simulink model "Load_Rate_Actuator"  (R2012b)
settings: Solver=ode4  StartTime=0.0  StopTime=2.999  FixedStep=1e-5  MaxStep=1e-3  MinStep=1e-4
undefined symbols (not defined in the file or in its folder): Acv, Aleak1, Aleak2, Aleak3, Aleak4, Aleak5, Aleakext, Aleakint, Ap, Ap_seal, Ar_seal, As_ehsv, Bkp_seal, Bp1, C, Cd, DeltaQ_ehsv, EHSV, EHSV_step, EHSVFreqTest, EHSVTest, ent_air, frictionstribeck_velocity, i_ehsv, K2_ehsv, K3_ehsv, K_Supply1, Ka1, Ki_ehsv, Kr_ehsv, ksi_ehsv, Kst, Kst_Enable, Kw_ehsv, L0, load_cmd, Lp_seal, Lr_seal, Mp1, P10, Pcvac, Pcvi, Pcvr, Ps0, Pt0, Ql_ehsv, R, rate_high, rate_low, Return_Pressure, Rho, seal_compression, seal_hardness, SealConstValue, SealType, Supply_Pressure, Temp, Theta0, V011, V021 ... (+10)
undefined symbols (not defined in the file): dpLVDT, ramLVDT, xvLVDT
libraries: simulink x2
(part 1 of 2)
settings Model: SimulationMode=accelerator  Creator=Charles  LastModifiedBy=hballest
settings SolverCC: InitialStep=1e-4
settings DataIOCC: LimitDataPoints=off  SaveFormat=StructureWithTime  DSMLogging=off  SaveTime=off
settings OptimizationCC: InitFltsAndDblsToZero=on
settings DebuggingCC: SaveWithParameterizedLinksMsg=none  InheritedTsInSrcMsg=none  FcnCallInpInsideContextMsg=UseLocalSettings  LoggingUnavailableSignals=none
settings ModelReferenceCC: UpdateModelReferenceTargets=IfOutOfDate
settings GRTTargetCC: TargetFcnLib=ansi_tfl_tmw.mat  CombineOutputUpdateFcns=off  GRTInterface=on

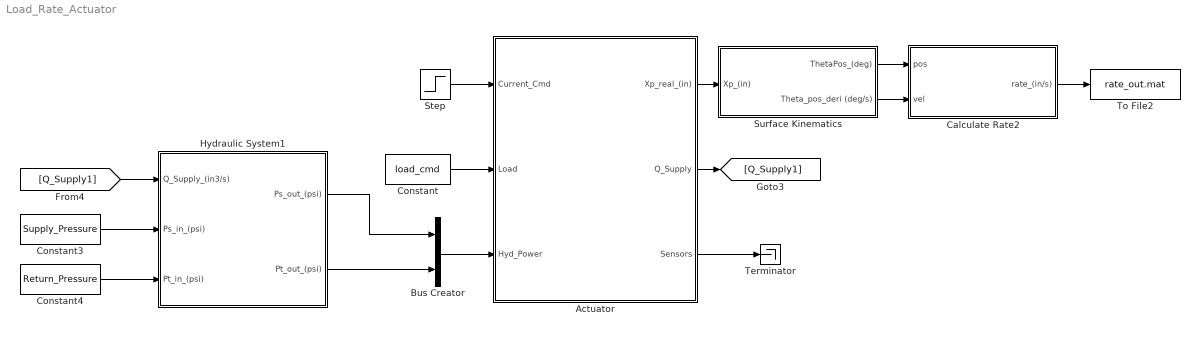
== system Load_Rate_Actuator ==
  Actuator : Subsystem
  Bus Creator : BusCreator  Inputs=2
  Calculate Rate2 : Subsystem
  Constant : Constant  Value=load_cmd
  Constant3 : Constant  Value=Supply_Pressure
  Constant4 : Constant  Value=Return_Pressure
  Hydraulic System1 : Subsystem
  Step : Step  Time=.5  After=EHSV_step.final  SampleTime=0
  Surface Kinematics : Subsystem
  Terminator : Terminator
  To File2 : ToFile  Filename=rate_out.mat  MatrixName=rate_out
  wires:
  Actuator/1(Xp_real_(in)) -> Surface Kinematics/1(Xp_(in))
  Constant3/1 -> Hydraulic System1/2(Ps_in_(psi))
  Constant4/1 -> Hydraulic System1/3(Pt_in_(psi))
  Hydraulic System1/1(Ps_out_(psi)) -> Bus Creator/1
  Hydraulic System1/2(Pt_out_(psi)) -> Bus Creator/2
  [Q_Supply1] -> Hydraulic System1/1(Q_Supply_(in3/s))
  Bus Creator/1 -> Actuator/3(Hyd_Power)
  Actuator/2(Q_Supply) -> [Q_Supply1]
  Actuator/3(Sensors) -> Terminator/1
  Constant/1 -> Actuator/2(Load)
  Step/1 -> Actuator/1(Current_Cmd)
  Surface Kinematics/1(ThetaPos_(deg)) -> Calculate Rate2/1(pos)
  Surface Kinematics/2(Theta_pos_deri (deg/s)) -> Calculate Rate2/2(vel)
  Calculate Rate2/1(rate_(in/s)) -> To File2/1

== system Load_Rate_Actuator/Actuator ==
  Current_Cmd : Inport
  Load : Inport  Port=2
  Hyd_Power : Inport  Port=3
  Cylinder Dynamics : Subsystem
  Sensors Dynamics : Subsystem
  Valves Dynamics : Subsystem
  Xp_real_(in) : Outport
  Q_Supply : Outport  Port=2
  Sensors : Outport  Port=3
  wires:
  Cylinder Dynamics/2(Xp) -> [Xp], Xp_real_(in)/1
  Load/1 -> Cylinder Dynamics/2(Load)
  Valves Dynamics/2(Q_Supply) -> Q_Supply/1
  Valves Dynamics/1(Q_Act) -> Cylinder Dynamics/1(Q_Act)
  Current_Cmd/1 -> Valves Dynamics/2(Currrent)
  Hyd_Power/1 -> Valves Dynamics/3(Hyd_Pwr)
  Cylinder Dynamics/1(P_Act) -> Valves Dynamics/1(P_Act)
  Cylinder Dynamics/3(Qacv) -> Valves Dynamics/4(Qacv)
  Valves Dynamics/3(Pt) -> Cylinder Dynamics/3(Pt)
  Valves Dynamics/4(Xv_(in)) -> [Xv]
  Cylinder Dynamics/4(dP) -> [dP]
  [Xp] -> Sensors Dynamics/1(Xp)
  [dP] -> Sensors Dynamics/2(dP)
  [Xv] -> Sensors Dynamics/3(Xv)
  Sensors Dynamics/1(Sensors) -> Sensors/1

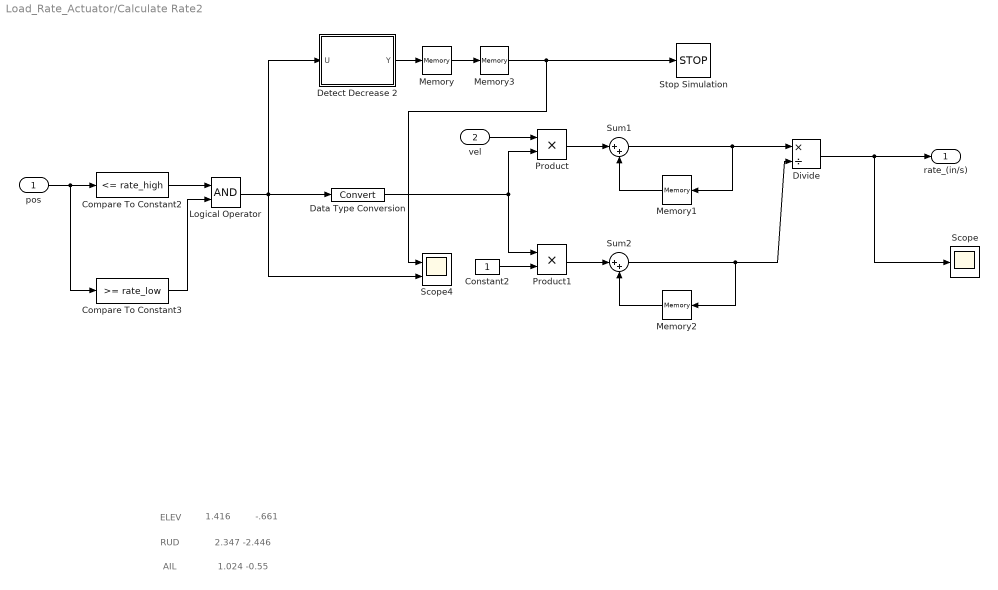
== system Load_Rate_Actuator/Calculate Rate2 ==
  note: 2.347 -2.446
  note: RUD
  note: ELEV
  note: -.661
  note: 1.416
  note: 1.024 -0.55
  note: AIL
  pos : Inport
  vel : Inport  Port=2
  Compare To Constant2 : simulink/Logic and Bit Operations/Compare To Constant  relop=<=  const=rate_high  OutDataTypeStr=boolean
  Compare To Constant3 : simulink/Logic and Bit Operations/Compare To Constant  relop=>=  const=rate_low  OutDataTypeStr=boolean
  Constant2 : Constant
  Data Type Conversion : DataTypeConversion
  Detect Decrease 2 : Subsystem
  Divide : Product  Inputs=*/
  Logical Operator : Logic  AllPortsSameDT=off  OutDataTypeStr=boolean
  Memory : Memory  X0=0.0
  Memory1 : Memory
  Memory2 : Memory  X0=0.0001
  Memory3 : Memory  X0=0.0
  Product : Product  RndMeth=Zero
  Product1 : Product  RndMeth=Zero
  Scope : Scope
      settings: SaveName=ScopeData5
  Scope4 : Scope  NumInputPorts=2
      settings: YMin=-5~-5  YMax=5~5  SaveName=ScopeData13
  Stop Simulation : Stop
  Sum1 : Sum  Inputs=|++
  Sum2 : Sum  Inputs=|++
  rate_(in/s) : Outport
  wires:
  pos/1 -> Compare To Constant2/1, Compare To Constant3/1
  Detect Decrease 2/1(Y) -> Memory/1
  Constant2/1 -> Product1/2
  Product1/1 -> Sum2/1
  Sum2/1 -> Memory2/1, Divide/2
  Memory2/1 -> Sum2/2
  Data Type Conversion/1 -> Product/2, Product1/1
  Compare To Constant3/1 -> Logical Operator/2
  Compare To Constant2/1 -> Logical Operator/1
  Sum1/1 -> Divide/1, Memory1/1
  Product/1 -> Sum1/1
  Memory1/1 -> Sum1/2
  vel/1 -> Product/1
  Logical Operator/1 -> Detect Decrease 2/1(U), Scope4/2, Data Type Conversion/1
  Memory/1 -> Memory3/1
  Memory3/1 -> Stop Simulation/1, Scope4/1
  Divide/1 -> Scope/1, rate_(in/s)/1

== system Load_Rate_Actuator/Hydraulic System1 ==
  Q_Supply_(in3/s) : Inport
  Ps_in_(psi) : Inport  Port=2
  Pt_in_(psi) : Inport  Port=3
  Aircraft Hydraulic Losses : Gain  Gain=K_Supply1
  Bus Selector : BusSelector  OutputSignals=Qs
  Fluid Inertia : TransferFcn  Denominator=[0.01 1]
  Sum1 : Sum  Inputs=|+-
  cis to gpm : Gain  Gain=0.25974
  Ps_out_(psi) : Outport
  Pt_out_(psi) : Outport  Port=2
  wires:
  Sum1/1 -> Ps_out_(psi)/1  "Ps"
  Aircraft Hydraulic Losses/1 -> Fluid Inertia/1
  Fluid Inertia/1 -> Sum1/2
  Pt_in_(psi)/1 -> Pt_out_(psi)/1  "Pt"
  Ps_in_(psi)/1 -> Sum1/1  "Ps"
  Q_Supply_(in3/s)/1 -> Bus Selector/1
  cis to gpm/1 -> Aircraft Hydraulic Losses/1
  Bus Selector/1 -> cis to gpm/1  "<Qs>"

== system Load_Rate_Actuator/Surface Kinematics ==
  Xp_(in) : Inport
  Derivative : Derivative
  Rad2Deg : Gain  Gain=180/pi  SaturateOnIntegerOverflow=on  OutDataTypeStr=Inherit: Same as input  ParamDataTypeStr=Inherit: Same as input
  Real Kinematics : Subsystem
  Terminator : Terminator
  ThetaPos_(deg) : Outport
  Theta_pos_deri (deg/s) : Outport  Port=2
  wires:
  Xp_(in)/1 -> Real Kinematics/1(Xp)
  Real Kinematics/1(Theta) -> Rad2Deg/1
  Rad2Deg/1 -> Derivative/1, ThetaPos_(deg)/1
  Real Kinematics/2(Reff) -> Terminator/1
  Derivative/1 -> Theta_pos_deri (deg/s)/1

== system Load_Rate_Actuator/Actuator/Cylinder Dynamics ==
  Q_Act : Inport
  Load : Inport  Port=2
  Pt : Inport  Port=3
  Bus Creator1 : BusCreator  Inputs=2
  Bus Creator3 : BusCreator  Inputs=2
  Bus Selector : BusSelector  OutputSignals=Q1,Q2
  Fluid Dynamics : Subsystem
  Piston Dynamics : Subsystem
  P_Act : Outport
  Xp : Outport  Port=2
  Qacv : Outport  Port=3
  dP : Outport  Port=4
  wires:
  Bus Creator3/1 -> P_Act/1
  Q_Act/1 -> Bus Selector/1
  Bus Selector/2 -> Fluid Dynamics/4(Q2)  "<Q2>"
  Piston Dynamics/1(Xp) -> [Xp], Xp/1
  Piston Dynamics/2(Xpdot) -> [Xpdot]  "Xpdot"
  [Xp] -> Fluid Dynamics/1(xp)
  [Xpdot] -> Fluid Dynamics/2(xpdot)
  Load/1 -> Piston Dynamics/3(FL)
  Bus Selector/1 -> Fluid Dynamics/3(Q1)  "<Q1>"
  Fluid Dynamics/2(P2) -> Piston Dynamics/2(Pr), Bus Creator3/2  "P2"
  Fluid Dynamics/1(P1) -> Piston Dynamics/1(Pe), Bus Creator3/1  "P1"
  Pt/1 -> Fluid Dynamics/5(Pt)
  Fluid Dynamics/3(Qacv1) -> Bus Creator1/1  "Qacv1"
  Fluid Dynamics/4(Qacv2) -> Bus Creator1/2  "Qacv2"
  Bus Creator1/1 -> Qacv/1
  Fluid Dynamics/5(dP) -> dP/1

== system Load_Rate_Actuator/Actuator/Sensors Dynamics ==
  Xp : Inport
  dP : Inport  Port=2
  Xv : Inport  Port=3
  Bus Creator : BusCreator  Inputs=3
  "Xp LVDT " : Subsystem
  "Xv LVDT " : Subsystem
  "dP LVDT " : Subsystem
  Sensors : Outport
  wires:
  dP/1 -> "dP LVDT "/1(dP_real)
  Xp/1 -> "Xp LVDT "/1(Xp_real)
  Xv/1 -> "Xv LVDT "/1(Xv_real)
  "Xv LVDT "/1(Xv_LVDT) -> Bus Creator/3  "Xv_mesured_(in)"
  "dP LVDT "/1(dP_LVDT) -> Bus Creator/2  "dP_mesured_(psi)"
  "Xp LVDT "/1(Xp_LVDT) -> Bus Creator/1  "Xp_mesured_(in)"
  Bus Creator/1 -> Sensors/1

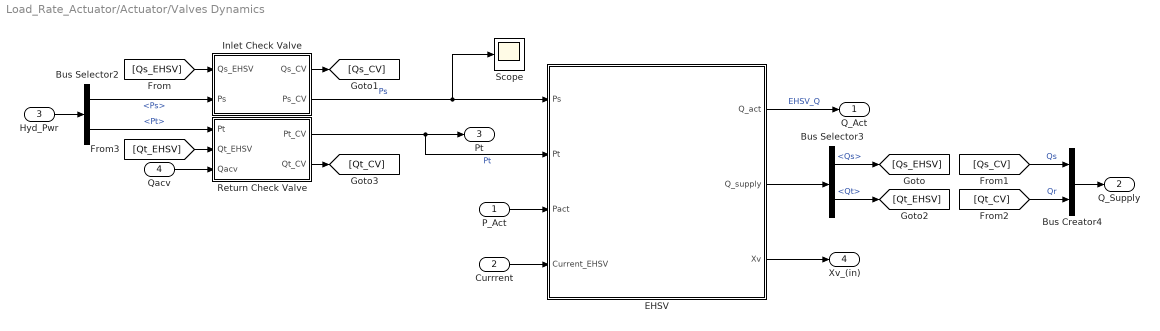
== system Load_Rate_Actuator/Actuator/Valves Dynamics ==
  P_Act : Inport
  Currrent : Inport  Port=2
  Hyd_Pwr : Inport  Port=3
  Qacv : Inport  Port=4
  Bus Creator4 : BusCreator  Inputs=2
  Bus Selector2 : BusSelector  OutputSignals=Ps,Pt
  Bus Selector3 : BusSelector  OutputSignals=Qs,Qt
  EHSV : Subsystem
  Inlet Check Valve : Subsystem
  Return Check Valve : Subsystem
  Scope : Scope
      settings: SaveName=ScopeData5
  Q_Act : Outport
  Q_Supply : Outport  Port=2
  Pt : Outport  Port=3
  Xv_(in) : Outport  Port=4
  wires:
  Hyd_Pwr/1 -> Bus Selector2/1
  EHSV/1(Q_act) -> Q_Act/1  "EHSV_Q"
  Bus Selector2/1 -> Inlet Check Valve/2(Ps)  "<Ps>"
  Bus Selector3/1 -> [Qs_EHSV]  "<Qs>"
  [Qs_EHSV] -> Inlet Check Valve/1(Qs_EHSV)
  Inlet Check Valve/1(Qs_CV) -> [Qs_CV]
  [Qs_CV] -> Bus Creator4/1  "Qs"
  Bus Creator4/1 -> Q_Supply/1
  Bus Selector2/2 -> Return Check Valve/1(Pt)  "<Pt>"
  Bus Selector3/2 -> [Qt_EHSV]  "<Qt>"
  [Qt_CV] -> Bus Creator4/2  "Qr"
  [Qt_EHSV] -> Return Check Valve/2(Qt_EHSV)
  Return Check Valve/2(Qt_CV) -> [Qt_CV]
  Qacv/1 -> Return Check Valve/3(Qacv)
  Currrent/1 -> EHSV/4(Current_EHSV)
  P_Act/1 -> EHSV/3(Pact)
  Inlet Check Valve/2(Ps_CV) -> Scope/1, EHSV/1(Ps)  "Ps"
  Return Check Valve/1(Pt_CV) -> EHSV/2(Pt), Pt/1  "Pt"
  EHSV/2(Q_supply) -> Bus Selector3/1
  EHSV/3(Xv) -> Xv_(in)/1

== system Load_Rate_Actuator/Calculate Rate2/Detect Decrease 2 ==
  note: Edge
  note: U(k)
  U : Inport
  FixPt Relational Operator : RelationalOperator  Operator=<  OutDataTypeStr=boolean  ZeroCross=off
  Memory : Memory  X0=0.0
  Y : Outport  InitialOutput=0
  wires:
  U/1 -> Memory/1, FixPt Relational Operator/1
  FixPt Relational Operator/1 -> Y/1
  Memory/1 -> FixPt Relational Operator/2  "U(k-1)"

== system Load_Rate_Actuator/Surface Kinematics/Real Kinematics ==
  Xp : Inport
  Bus Creator : BusCreator
  Bus Selector2 : BusSelector  OutputSignals=C,R,L
  Bus Selector3 : BusSelector  OutputSignals=L,C,R
  Bus Selector4 : BusSelector  OutputSignals=Theta0
  Bus Selector5 : BusSelector  OutputSignals=C
  Constant : Constant  Value=L0
  Constant1 : Constant  Value=R
  Constant2 : Constant  Value=C
  Constant3 : Constant  Value=Theta0
  Law of cosines Get angle : Fcn  Expr=acos((u(1)^2+u(2)^2-u(3)^2)/(2*u(1)*u(2)))
  Law of cosines Get angle1 : Fcn  Expr=acos((u(1)^2+u(2)^2-u(3)^2)/(2*u(1)*u(2)))
  Mux1 : Mux  Inputs=3
  Mux2 : Mux  Inputs=3
  Product : Product  RndMeth=Zero
  Sum1 : Sum  Inputs=++|
  Sum4 : Sum  Inputs=|+-
  Trigonometric Function : Trigonometry
  Theta : Outport
  Reff : Outport  Port=2
  wires:
  Mux2/1 -> Law of cosines Get angle1/1
  Bus Selector2/1 -> Mux2/1  "<C>"
  Bus Selector2/2 -> Mux2/2  "<R>"
  Law of cosines Get angle1/1 -> Sum4/1  "theta"
  Bus Selector4/1 -> Sum4/2  "<Theta0>"
  Sum4/1 -> Theta/1
  Xp/1 -> Sum1/1  "Xp"
  Constant/1 -> Sum1/2  "L0"
  Sum1/1 -> Bus Creator/1  "L"
  Constant2/1 -> Bus Creator/2  "C"
  Constant1/1 -> Bus Creator/3  "R"
  Constant3/1 -> Bus Creator/4  "Theta0"
  Mux1/1 -> Law of cosines Get angle/1
  Law of cosines Get angle/1 -> Trigonometric Function/1  "alfa"
  Bus Selector3/1 -> Mux1/1  "<L>"
  Bus Selector3/2 -> Mux1/2  "<C>"
  Bus Selector3/3 -> Mux1/3  "<R>"
  Product/1 -> Reff/1  "Reff"
  Bus Selector5/1 -> Product/1  "<C>"
  Trigonometric Function/1 -> Product/2
  Bus Selector2/3 -> Mux2/3  "<L>"
  Bus Creator/1 -> Bus Selector3/1, Bus Selector5/1, Bus Selector2/1, Bus Selector4/1

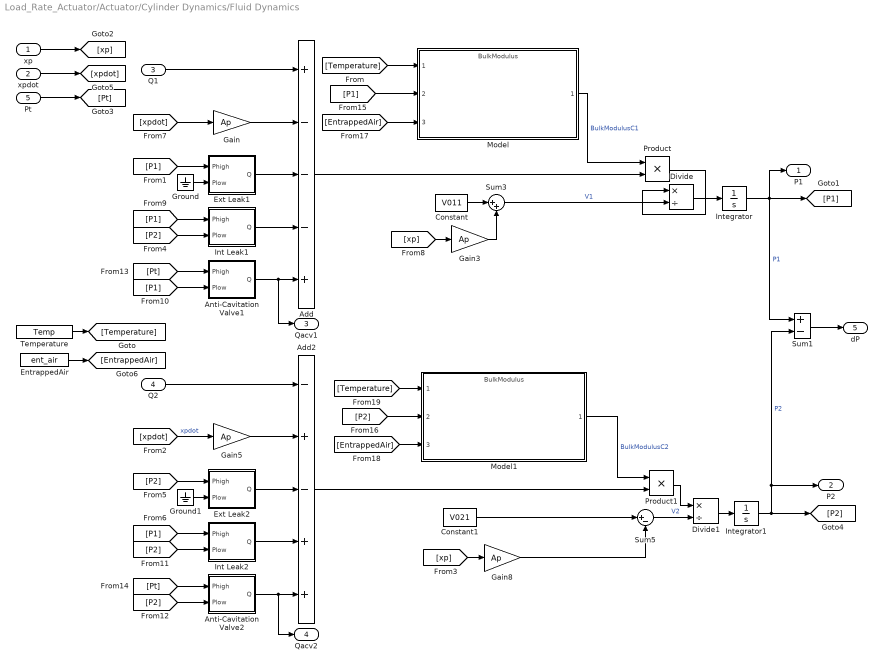
== system Load_Rate_Actuator/Actuator/Cylinder Dynamics/Fluid Dynamics ==
  xp : Inport
  xpdot : Inport  Port=2
  Q1 : Inport  Port=3
  Q2 : Inport  Port=4
  Pt : Inport  Port=5
  Add : Sum  Inputs=+---+
  Add2 : Sum  Inputs=-+-++
  Anti-Cavitation Valve1 : Subsystem
  Anti-Cavitation Valve2 : Subsystem
  Constant : Constant  Value=V011
  Constant1 : Constant  Value=V021
  Divide : Product  Inputs=*/
  Divide1 : Product  Inputs=*/
  EntrappedAir : Constant  Value=ent_air
  Ext Leak1 : Subsystem
  Ext Leak2 : Subsystem
  Gain{,3,5,8} (4 alike) : Gain  Gain=Ap
  Ground : Ground
  Ground1 : Ground
  Int Leak1 : Subsystem
  Int Leak2 : Subsystem
  Integrator : Integrator  InitialCondition=P10
  Integrator1 : Integrator  InitialCondition=P10
  Model : ModelReference  ModelNameDialog=BulkModulus  SimulationMode=Normal  ModelReferenceVersion=1.7  CopyOfModelName=BulkModulus  DefaultDataLogging=off
  Model1 : ModelReference  ModelNameDialog=BulkModulus  SimulationMode=Normal  ModelReferenceVersion=1.7  CopyOfModelName=BulkModulus  DefaultDataLogging=off
  Product : Product  RndMeth=Zero
  Product1 : Product  RndMeth=Zero
  Sum1 : Sum  Inputs=+-
  Sum3 : Sum  Inputs=|++
  Sum5 : Sum  Inputs=|+-
  Temperature : Constant  Value=Temp
  P1 : Outport
  P2 : Outport  Port=2
  Qacv1 : Outport  Port=3
  Qacv2 : Outport  Port=4
  dP : Outport  Port=5
  wires:
  Q1/1 -> Add/1
  Q2/1 -> Add2/1
  [xpdot] -> Gain5/1  "xpdot"
  [xp] -> Gain8/1
  Int Leak2/1(Q) -> Add2/4
  Divide1/1 -> Integrator1/1
  Sum5/1 -> Divide1/2  "V2"
  Gain8/1 -> Sum5/2
  Constant1/1 -> Sum5/1
  Integrator1/1 -> [P2], Sum1/2, P2/1  "P2"
  Ext Leak2/1(Q) -> Add2/3
  Gain5/1 -> Add2/2
  Int Leak1/1(Q) -> Add/4
  Divide/1 -> Integrator/1
  Sum3/1 -> Divide/2  "V1"
  Gain3/1 -> Sum3/2
  Constant/1 -> Sum3/1
  Integrator/1 -> Sum1/1, [P1], P1/1  "P1"
  Ext Leak1/1(Q) -> Add/3
  Add/1 -> Product/2
  Gain/1 -> Add/2
  [P1] -> Ext Leak1/1(Phigh)
  [P2] -> Ext Leak2/1(Phigh)
  xpdot/1 -> [xpdot]
  [xpdot] -> Gain/1
  xp/1 -> [xp]
  [xp] -> Gain3/1
  [P2] -> Int Leak1/2(Plow)
  Ground/1 -> Ext Leak1/2(Plow)
  Ground1/1 -> Ext Leak2/2(Plow)
  [P1] -> Int Leak2/1(Phigh)
  [Pt] -> Anti-Cavitation Valve1/1(Phigh)
  [P1] -> Anti-Cavitation Valve1/2(Plow)
  [P1] -> Int Leak1/1(Phigh)
  Anti-Cavitation Valve1/1(Q) -> Add/5, Qacv1/1
  [P2] -> Int Leak2/2(Plow)
  Anti-Cavitation Valve2/1(Q) -> Add2/5, Qacv2/1
  [Pt] -> Anti-Cavitation Valve2/1(Phigh)
  [P2] -> Anti-Cavitation Valve2/2(Plow)
  Pt/1 -> [Pt]
  Product/1 -> Divide/1
  [P1] -> Model/2
  Model/1 -> Product/1  "BulkModulusC1"
  Product1/1 -> Divide1/1
  Model1/1 -> Product1/1  "BulkModulusC2"
  Add2/1 -> Product1/2
  [P2] -> Model1/2
  Temperature/1 -> [Temperature]
  EntrappedAir/1 -> [EntrappedAir]
  [Temperature] -> Model/1
  [EntrappedAir] -> Model/3
  [EntrappedAir] -> Model1/3
  [Temperature] -> Model1/1
  Sum1/1 -> dP/1

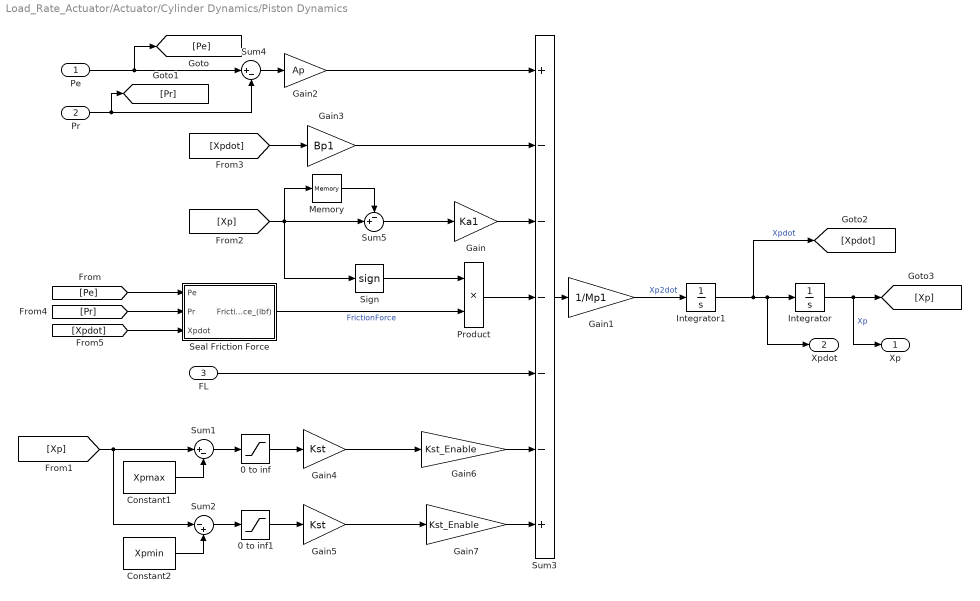
== system Load_Rate_Actuator/Actuator/Cylinder Dynamics/Piston Dynamics ==
  Pe : Inport
  Pr : Inport  Port=2
  FL : Inport  Port=3
  0 to inf : Saturate  UpperLimit=inf  LowerLimit=0
  0 to inf1 : Saturate  UpperLimit=inf  LowerLimit=0
  Constant1 : Constant  Value=Xpmax
  Constant2 : Constant  Value=Xpmin
  Gain : Gain  Gain=Ka1
  Gain1 : Gain  Gain=1/Mp1
  Gain2 : Gain  Gain=Ap
  Gain3 : Gain  Gain=Bp1
  Gain4 : Gain  Gain=Kst
  Gain5 : Gain  Gain=Kst
  Gain6 : Gain  Gain=Kst_Enable
  Gain7 : Gain  Gain=Kst_Enable
  Integrator : Integrator  InitialCondition=Xp_init
  Integrator1 : Integrator  InitialCondition=0.0001
  Memory : Memory
  Product : Product  RndMeth=Zero
  Seal Friction Force : Subsystem
  Sign : Signum
  Sum1 : Sum  Inputs=|+-
  Sum2 : Sum  Inputs=|-+
  Sum3 : Sum  Inputs=+-----+
  Sum4 : Sum  Inputs=|+-
  Sum5 : Sum  Inputs=-+|
  Xp : Outport
  Xpdot : Outport  Port=2
  wires:
  Sum3/1 -> Gain1/1
  Gain1/1 -> Integrator1/1  "Xp2dot"
  Integrator1/1 -> Integrator/1, Xpdot/1, [Xpdot]  "Xpdot"
  Integrator/1 -> [Xp], Xp/1  "Xp"
  [Xp] -> Sign/1, Sum5/2, Memory/1
  Pe/1 -> [Pe], Sum4/1
  Sum4/1 -> Gain2/1
  Gain2/1 -> Sum3/1
  [Xpdot] -> Gain3/1
  Gain3/1 -> Sum3/2
  Gain/1 -> Sum3/3
  FL/1 -> Sum3/5
  Sum1/1 -> 0 to inf/1
  0 to inf/1 -> Gain4/1
  Constant2/1 -> Sum2/2
  Sign/1 -> Product/1
  Product/1 -> Sum3/4
  [Xp] -> Sum1/1, Sum2/1
  Gain4/1 -> Gain6/1
  Sum2/1 -> 0 to inf1/1
  0 to inf1/1 -> Gain5/1
  Gain5/1 -> Gain7/1
  Constant1/1 -> Sum1/2
  Memory/1 -> Sum5/1
  Sum5/1 -> Gain/1
  Seal Friction Force/1(FrictionForce_(lbf)) -> Product/2  "FrictionForce"
  Pr/1 -> [Pr], Sum4/2
  [Pr] -> Seal Friction Force/2(Pr)
  [Pe] -> Seal Friction Force/1(Pe)
  Gain6/1 -> Sum3/6
  Gain7/1 -> Sum3/7
  [Xpdot] -> Seal Friction Force/3(Xpdot)

== system Load_Rate_Actuator/Actuator/Sensors Dynamics/Xp LVDT  ==
  Xp_real : Inport
  LVDT : Subsystem  mask{band=ramLVDT.Bandwidth, range=ramLVDT.Range, lvdt_error=ramLVDT.Error, hyst=ramLVDT.Hysteresis}
      mask prompts: band "LVDT Bandwdidth"; range "LVDT Range ([min middle max])"; lvdt_error "LVDT error"; hyst "LVDT Hysteresis"
  Xp_LVDT : Outport
  wires:
  Xp_real/1 -> LVDT/1(Sensor In)
  LVDT/1(SensorOut) -> Xp_LVDT/1

== system Load_Rate_Actuator/Actuator/Sensors Dynamics/Xv LVDT  ==
  Xv_real : Inport
  LVDT1 : Subsystem  mask{band=xvLVDT.Bandwidth, range=xvLVDT.Range, lvdt_error=xvLVDT.Error, hyst=xvLVDT.Hysteresis}
      mask prompts: band "LVDT Bandwdidth (Hz)"; range "LVDT Range ([min middle max])"; lvdt_error "LVDT error"; hyst "LVDT Hysteresis (%)"
  Xv_LVDT : Outport
  wires:
  Xv_real/1 -> LVDT1/1(Sensor In)
  LVDT1/1(SensorOut) -> Xv_LVDT/1

== system Load_Rate_Actuator/Actuator/Sensors Dynamics/dP LVDT  ==
  dP_real : Inport
  LVDT1 : Subsystem  mask{band=dpLVDT.Bandwidth, range=dpLVDT.Range, lvdt_error=dpLVDT.Error, hyst=dpLVDT.Hysteresis}
      mask prompts: band "LVDT Bandwdidth (Hz)"; range "LVDT Range ([min middle max])"; lvdt_error "LVDT error"; hyst "LVDT Hysteresis (%)"
  dP_LVDT : Outport
  wires:
  dP_real/1 -> LVDT1/1(Sensor In)
  LVDT1/1(SensorOut) -> dP_LVDT/1

== system Load_Rate_Actuator/Actuator/Valves Dynamics/EHSV ==
  Ps : Inport
  Pt : Inport  Port=2
  Pact : Inport  Port=3
  Current_EHSV : Inport  Port=4
  Bus Selector1 : BusSelector  OutputSignals=P1,P2
  Derivative : Derivative
  EHSV 1st Stage : Subsystem
  EHSV 2nd Stage : Subsystem
  EHSV Test : Subsystem
  EHSV Test1 : Subsystem
  EHSV Test2 : Subsystem
  EHSV Test3 : Subsystem
  EHSV input : Subsystem
  Scope : Scope
  Scope1 : Scope  NumInputPorts=2
      settings: YMin=-5~-5  YMax=5~5  SaveName=ScopeData4
  Q_act : Outport
  Q_supply : Outport  Port=2
  Xv : Outport  Port=3
  wires:
  Bus Selector1/1 -> EHSV Test/1(In1)  "<P1>"
  Bus Selector1/2 -> EHSV Test1/1(In1)  "<P2>"
  EHSV 1st Stage/1(Xv) -> Derivative/1, Xv/1, EHSV 2nd Stage/5(Xv)  "Xv"
  EHSV Test/1(Out1) -> EHSV 2nd Stage/3(P1)  "P1"
  EHSV Test1/1(Out1) -> EHSV 2nd Stage/4(P2)  "P2"
  Pt/1 -> EHSV Test3/1(In1)
  EHSV 2nd Stage/1(Q) -> Q_act/1  "EHSV_Q"
  Ps/1 -> EHSV Test2/1(In1)
  Current_EHSV/1 -> EHSV input/1(CurrentCmd)
  Pact/1 -> Bus Selector1/1
  EHSV 2nd Stage/2(Q_Supply) -> Q_supply/1
  EHSV Test2/1(Out1) -> EHSV 2nd Stage/1(Ps)  "Ps"
  EHSV Test3/1(Out1) -> EHSV 2nd Stage/2(Pt)  "Pt"
  EHSV input/1(EHSV_current) -> EHSV 1st Stage/1(i)  "EHSV_current_cmd"
  EHSV 2nd Stage/3(Q_leak_EHV) -> Scope/1  "Qleak_EHSV"
  Derivative/1 -> Scope1/1, Scope1/2

== system Load_Rate_Actuator/Actuator/Valves Dynamics/Inlet Check Valve ==
  Qs_EHSV : Inport
  Ps : Inport  Port=2
  Divide : Product  Inputs=*/
  EntrappedAir : Constant  Value=ent_air
  Inlet Check Valve Flow : Subsystem
  Integrator : Integrator  InitialCondition=Ps0
  Model : ModelReference  ModelNameDialog=BulkModulus  SimulationMode=Normal  ModelReferenceVersion=1.7  CopyOfModelName=BulkModulus  DefaultDataLogging=off
  Product : Product  RndMeth=Zero
  Sum : Sum  Inputs=-+|
  Temperature : Constant  Value=Temp
  Vcv : Constant  Value=Vcv
  Qs_CV : Outport
  Ps_CV : Outport  Port=2
  wires:
  Inlet Check Valve Flow/1(Q) -> Sum/2, Qs_CV/1
  Qs_EHSV/1 -> Sum/1
  Integrator/1 -> Inlet Check Valve Flow/2(P2), Ps_CV/1
  Sum/1 -> Product/2
  Product/1 -> Integrator/1
  Temperature/1 -> [Temperature]
  EntrappedAir/1 -> [EntrappedAir]
  Ps/1 -> Model/2, Inlet Check Valve Flow/1(P1)
  [Temperature] -> Model/1
  [EntrappedAir] -> Model/3
  Divide/1 -> Product/1
  Model/1 -> Divide/1
  Vcv/1 -> Divide/2

== system Load_Rate_Actuator/Actuator/Valves Dynamics/Return Check Valve ==
  Pt : Inport
  Qt_EHSV : Inport  Port=2
  Qacv : Inport  Port=3
  Bus Selector1 : BusSelector  OutputSignals=Qacv1,Qacv2
  Divide : Product  Inputs=*/
  EntrappedAir : Constant  Value=ent_air
  Integrator : Integrator  InitialCondition=Pt0
  Model : ModelReference  ModelNameDialog=BulkModulus  SimulationMode=Normal  ModelReferenceVersion=1.7  CopyOfModelName=BulkModulus  DefaultDataLogging=off
  Product : Product  RndMeth=Zero
  Return Check Valve Flow : Subsystem
  Sum : Sum  Inputs=+--
  Sum1 : Sum  Inputs=++|
  Temperature : Constant  Value=Temp
  Vcv : Constant  Value=Vcv
  Pt_CV : Outport
  Qt_CV : Outport  Port=2
  wires:
  Sum/1 -> Product/2
  Integrator/1 -> Return Check Valve Flow/2(P2), Pt_CV/1
  Pt/1 -> Model/2, Return Check Valve Flow/1(P1)
  Qt_EHSV/1 -> Sum/1
  Return Check Valve Flow/1(Q) -> Qt_CV/1, Sum/2
  Product/1 -> Integrator/1
  Qacv/1 -> Bus Selector1/1
  Bus Selector1/1 -> Sum1/1  "<Qacv1>"
  Bus Selector1/2 -> Sum1/2  "<Qacv2>"
  Sum1/1 -> Sum/3
  Temperature/1 -> [Temperature]
  EntrappedAir/1 -> [EntrappedAir]
  [Temperature] -> Model/1
  [EntrappedAir] -> Model/3
  Divide/1 -> Product/1
  Model/1 -> Divide/1
  Vcv/1 -> Divide/2

== system Load_Rate_Actuator/Actuator/Cylinder Dynamics/Fluid Dynamics/Anti-Cavitation Valve1 ==
  Phigh : Inport
  Plow : Inport  Port=2
  Abs : Abs
  Constant : Constant  Value=Acv*sqrt(2/Rho)
  Constant1 : Constant  Value=Pcvac
  Gain : Gain  Gain=Cd/Pcvac
  Math Function : Math  Operator=sqrt  SaturateOnIntegerOverflow=on
  Product : Product  RndMeth=Zero
  Product1 : Product  RndMeth=Zero
  Product2 : Product  RndMeth=Zero
  Saturation : Saturate  UpperLimit=Cd  LowerLimit=0
  Sign : Signum
  Sum : Sum  Inputs=|+-
  Sum1 : Sum  Inputs=|+-
  Q : Outport
  wires:
  Phigh/1 -> Sum/1
  Plow/1 -> Sum/2
  Sum/1 -> Sum1/1, Abs/1, Sign/1
  Constant1/1 -> Sum1/2
  Sum1/1 -> Gain/1
  Gain/1 -> Saturation/1
  Saturation/1 -> Product/1
  Constant/1 -> Product/2
  Abs/1 -> Math Function/1
  Sign/1 -> Product1/1
  Math Function/1 -> Product1/2
  Product1/1 -> Product2/1
  Product/1 -> Product2/2
  Product2/1 -> Q/1

== system Load_Rate_Actuator/Actuator/Cylinder Dynamics/Fluid Dynamics/Anti-Cavitation Valve2 ==
  Phigh : Inport
  Plow : Inport  Port=2
  Abs : Abs
  Constant : Constant  Value=Acv*sqrt(2/Rho)
  Constant1 : Constant  Value=Pcvac
  Gain : Gain  Gain=Cd/Pcvac
  Math Function : Math  Operator=sqrt  SaturateOnIntegerOverflow=on
  Product : Product  RndMeth=Zero
  Product1 : Product  RndMeth=Zero
  Product2 : Product  RndMeth=Zero
  Saturation : Saturate  UpperLimit=Cd  LowerLimit=0
  Sign : Signum
  Sum : Sum  Inputs=|+-
  Sum1 : Sum  Inputs=|+-
  Q : Outport
  wires:
  Product2/1 -> Q/1
  Product/1 -> Product2/2
  Product1/1 -> Product2/1
  Math Function/1 -> Product1/2
  Sign/1 -> Product1/1
  Abs/1 -> Math Function/1
  Constant/1 -> Product/2
  Saturation/1 -> Product/1
  Gain/1 -> Saturation/1
  Sum1/1 -> Gain/1
  Constant1/1 -> Sum1/2
  Sum/1 -> Sign/1, Abs/1, Sum1/1
  Plow/1 -> Sum/2
  Phigh/1 -> Sum/1

== system Load_Rate_Actuator/Actuator/Cylinder Dynamics/Fluid Dynamics/Ext Leak1 ==
  Phigh : Inport
  Plow : Inport  Port=2
  Abs : Abs
  Constant : Constant  Value=Cd*sqrt(2/Rho)
  Constant3 : Constant  Value=Aleakext
  Math Function : Math  Operator=sqrt  SaturateOnIntegerOverflow=on
  Product : Product  RndMeth=Zero
  Product1 : Product  RndMeth=Zero
  Product3 : Product  RndMeth=Zero
  Sign : Signum
  Sum : Sum  Inputs=|+-
  Q : Outport
  wires:
  Phigh/1 -> Sum/1
  Sum/1 -> Abs/1, Sign/1
  Abs/1 -> Math Function/1
  Sign/1 -> Product/1
  Math Function/1 -> Product/2
  Constant/1 -> Product1/2
  Product/1 -> Product1/1
  Constant3/1 -> Product3/2  "Atot"
  Product1/1 -> Product3/1
  Product3/1 -> Q/1
  Plow/1 -> Sum/2

== system Load_Rate_Actuator/Actuator/Cylinder Dynamics/Fluid Dynamics/Ext Leak2 ==
  Phigh : Inport
  Plow : Inport  Port=2
  Abs : Abs
  Constant : Constant  Value=Cd*sqrt(2/Rho)
  Constant3 : Constant  Value=Aleakext
  Math Function : Math  Operator=sqrt  SaturateOnIntegerOverflow=on
  Product : Product  RndMeth=Zero
  Product1 : Product  RndMeth=Zero
  Product3 : Product  RndMeth=Zero
  Sign : Signum
  Sum : Sum  Inputs=|+-
  Q : Outport
  wires:
  Plow/1 -> Sum/2
  Product3/1 -> Q/1
  Product1/1 -> Product3/1
  Constant3/1 -> Product3/2  "Atot"
  Product/1 -> Product1/1
  Constant/1 -> Product1/2
  Math Function/1 -> Product/2
  Sign/1 -> Product/1
  Abs/1 -> Math Function/1
  Sum/1 -> Sign/1, Abs/1
  Phigh/1 -> Sum/1

== system Load_Rate_Actuator/Actuator/Cylinder Dynamics/Fluid Dynamics/Int Leak1 ==
  Phigh : Inport
  Plow : Inport  Port=2
  Abs : Abs
  Constant : Constant  Value=Cd*sqrt(2/Rho)
  Constant3 : Constant  Value=Aleakint
  Math Function : Math  Operator=sqrt  SaturateOnIntegerOverflow=on
  Product : Product  RndMeth=Zero
  Product1 : Product  RndMeth=Zero
  Product3 : Product  RndMeth=Zero
  Sign : Signum
  Sum : Sum  Inputs=|+-
  Q : Outport
  wires:
  Plow/1 -> Sum/2
  Product3/1 -> Q/1
  Product1/1 -> Product3/1
  Constant3/1 -> Product3/2  "Atot"
  Product/1 -> Product1/1
  Constant/1 -> Product1/2
  Math Function/1 -> Product/2
  Sign/1 -> Product/1
  Abs/1 -> Math Function/1
  Sum/1 -> Sign/1, Abs/1
  Phigh/1 -> Sum/1

== system Load_Rate_Actuator/Actuator/Cylinder Dynamics/Fluid Dynamics/Int Leak2 ==
  Phigh : Inport
  Plow : Inport  Port=2
  Abs : Abs
  Constant : Constant  Value=Cd*sqrt(2/Rho)
  Constant3 : Constant  Value=Aleakint
  Math Function : Math  Operator=sqrt  SaturateOnIntegerOverflow=on
  Product : Product  RndMeth=Zero
  Product1 : Product  RndMeth=Zero
  Product3 : Product  RndMeth=Zero
  Sign : Signum
  Sum : Sum  Inputs=|+-
  Q : Outport
  wires:
  Phigh/1 -> Sum/1
  Sum/1 -> Abs/1, Sign/1
  Abs/1 -> Math Function/1
  Sign/1 -> Product/1
  Math Function/1 -> Product/2
  Constant/1 -> Product1/2
  Product/1 -> Product1/1
  Constant3/1 -> Product3/2  "Atot"
  Product1/1 -> Product3/1
  Product3/1 -> Q/1
  Plow/1 -> Sum/2

== system Load_Rate_Actuator/Actuator/Cylinder Dynamics/Piston Dynamics/Seal Friction Force ==
  Pe : Inport
  Pr : Inport  Port=2
  Xpdot : Inport  Port=3
  Constant : Constant  Value=SealType
  Constant3 : Constant  Value=SealConstValue
  Constant4 : Constant  Value=0
  Force friction 2 Rod backup + scrapper seal : Subsystem
  Force friction Piston+rod extension : Subsystem
  Force friction Piston+rod retraction : Subsystem
  Gain6 : Gain  Gain=Bkp_seal
  Product1 : Product  RndMeth=Zero
  Seal Friction type : MultiPortSwitch
  Stribeck effect : Subsystem
  Sum6 : Sum  Inputs=+++
  FrictionForce_(lbf) : Outport
  wires:
  Constant4/1 -> Force friction 2 Rod backup + scrapper seal/1(Pressure)
  Force friction Piston+rod extension/1(Ffriction) -> Sum6/1
  Force friction Piston+rod retraction/1(Ffriction) -> Sum6/2
  Force friction 2 Rod backup + scrapper seal/1(Ffriction) -> Gain6/1
  Gain6/1 -> Sum6/3
  Pe/1 -> Force friction Piston+rod extension/1(Pressure)
  Pr/1 -> Force friction Piston+rod retraction/1(Pressure)
  Product1/1 -> Seal Friction type/3
  Sum6/1 -> Product1/1, Seal Friction type/2
  Constant/1 -> Seal Friction type/1
  Seal Friction type/1 -> FrictionForce_(lbf)/1
  Constant3/1 -> Seal Friction type/4
  Xpdot/1 -> Stribeck effect/1(Xp)
  Stribeck effect/1(Stribeck factor) -> Product1/2

== system Load_Rate_Actuator/Actuator/Sensors Dynamics/Xp LVDT /LVDT ==
  Sensor In : Inport
  " Pos Error1" : Lookup_n-D  NumberOfTableDimensions=1  BreakpointsForDimension1=[range(1) range(2) range(3)]  Table=[lvdt_error lvdt_error*0.4 lvdt_error]  RndMeth=Simplest  InputSameDT=on
  Backlash : Backlash  BacklashWidth=(range(3)-range(2))*hyst/100
  LVDT Dynamics1 : TransferFcn  Numerator=[band]  Denominator=[1 band]
  Random1 : RandomNumber  Mean=1  Variance=10
  Sum2 : Sum  Inputs=|++
  Sum3 : Sum  Inputs=|+-
  Switch1 : Switch  Threshold=1
  SensorOut : Outport
  wires:
  [LVDTerror2] -> Sum3/2
  Switch1/1 -> LVDT Dynamics1/1
  Sum2/1 -> Switch1/1
  Sensor In/1 -> Sum2/1, Sum3/1, " Pos Error1"/1
  Random1/1 -> Switch1/2
  [LVDTerror2] -> Sum2/2
  Sum3/1 -> Switch1/3
  " Pos Error1"/1 -> [LVDTerror2]
  LVDT Dynamics1/1 -> Backlash/1
  Backlash/1 -> SensorOut/1

== system Load_Rate_Actuator/Actuator/Sensors Dynamics/Xv LVDT /LVDT1 ==
  Sensor In : Inport
  " Pos Error1" : Lookup_n-D  NumberOfTableDimensions=1  BreakpointsForDimension1=[range(1) range(2) range(3)]  Table=[lvdt_error lvdt_error*0.4 lvdt_error]  RndMeth=Simplest  InputSameDT=on
  Backlash : Backlash  BacklashWidth=(range(3)-range(2))*hyst/100
  LVDT Dynamics1 : TransferFcn  Numerator=[band]  Denominator=[1 band]
  Random1 : RandomNumber  Mean=1  Variance=10
  Sum2 : Sum  Inputs=|++
  Sum3 : Sum  Inputs=|+-
  Switch1 : Switch  Threshold=1
  SensorOut : Outport
  wires:
  [LVDTerror2] -> Sum3/2
  Switch1/1 -> LVDT Dynamics1/1
  Sum2/1 -> Switch1/1
  Sensor In/1 -> Sum2/1, Sum3/1, " Pos Error1"/1
  Random1/1 -> Switch1/2
  [LVDTerror2] -> Sum2/2
  Sum3/1 -> Switch1/3
  " Pos Error1"/1 -> [LVDTerror2]
  LVDT Dynamics1/1 -> Backlash/1
  Backlash/1 -> SensorOut/1

== system Load_Rate_Actuator/Actuator/Sensors Dynamics/dP LVDT /LVDT1 ==
  Sensor In : Inport
  " Pos Error1" : Lookup_n-D  NumberOfTableDimensions=1  BreakpointsForDimension1=[range(1) range(2) range(3)]  Table=[lvdt_error lvdt_error*0.4 lvdt_error]  RndMeth=Simplest  InputSameDT=on
  Backlash : Backlash  BacklashWidth=(range(3)-range(2))*hyst/100
  LVDT Dynamics1 : TransferFcn  Numerator=[band]  Denominator=[1 band]
  Random1 : RandomNumber  Mean=1  Variance=10
  Sum2 : Sum  Inputs=|++
  Sum3 : Sum  Inputs=|+-
  Switch1 : Switch  Threshold=1
  SensorOut : Outport
  wires:
  [LVDTerror2] -> Sum3/2
  Switch1/1 -> LVDT Dynamics1/1
  Sum2/1 -> Switch1/1
  Sensor In/1 -> Sum2/1, Sum3/1, " Pos Error1"/1
  Random1/1 -> Switch1/2
  [LVDTerror2] -> Sum2/2
  Sum3/1 -> Switch1/3
  " Pos Error1"/1 -> [LVDTerror2]
  LVDT Dynamics1/1 -> Backlash/1
  Backlash/1 -> SensorOut/1

== system Load_Rate_Actuator/Actuator/Valves Dynamics/EHSV/EHSV 1st Stage ==
  i : Inport
  Add : Sum  Inputs=|+-
  Armature flapper : TransferFcn  Numerator=[1/Kr_ehsv]  Denominator=[1/(w_n_ehsv^2) 2*ksi_ehsv/w_n_ehsv 1]
  EHSV 1st stage test : TransferFcn  Numerator=[.001852*730^2]  Denominator=[1 2*0.4*730 730^2]
  Feedback wire : Gain  Gain=Kw_ehsv
  Flapper displacement at nozzles : Saturate  UpperLimit=xf_ehsv  LowerLimit=-xf_ehsv
  Hydraulic Amplifier : Gain  Gain=K2_ehsv
  "Hydraulic Amplifier Differential flow " : Saturate  UpperLimit=DeltaQ_ehsv  LowerLimit=-DeltaQ_ehsv
  Scope : Scope  NumInputPorts=2
      settings: TimeRange=2.999  YMin=-5~-5  YMax=5~5  SaveName=ScopeData3
  Servovalve control flow : Saturate  UpperLimit=Ql_ehsv  LowerLimit=-Ql_ehsv
  Spool : TransferFcn  Denominator=[As_ehsv 0]
  Spool displacement : Saturate  UpperLimit=xs_ehsv  LowerLimit=-xs_ehsv
  Spool Flow Gain : Gain  Gain=K3_ehsv
  Terminator : Terminator
  Torque motor : Gain  Gain=Ki_ehsv
  Torque motor current : Saturate  UpperLimit=i_ehsv  LowerLimit=-i_ehsv
  Xv : Outport
  wires:
  Torque motor/1 -> Add/1
  Feedback wire/1 -> Add/2
  i/1 -> EHSV 1st stage test/1, Torque motor current/1
  Armature flapper/1 -> Flapper displacement at nozzles/1
  Spool/1 -> Scope/1, Spool displacement/1
  Hydraulic Amplifier/1 -> "Hydraulic Amplifier Differential flow "/1
  Add/1 -> Armature flapper/1
  Flapper displacement at nozzles/1 -> Hydraulic Amplifier/1
  "Hydraulic Amplifier Differential flow "/1 -> Spool/1
  Spool displacement/1 -> Spool Flow Gain/1, Xv/1, Feedback wire/1
  Torque motor current/1 -> Torque motor/1
  Spool Flow Gain/1 -> Servovalve control flow/1
  Servovalve control flow/1 -> Terminator/1
  EHSV 1st stage test/1 -> Scope/2

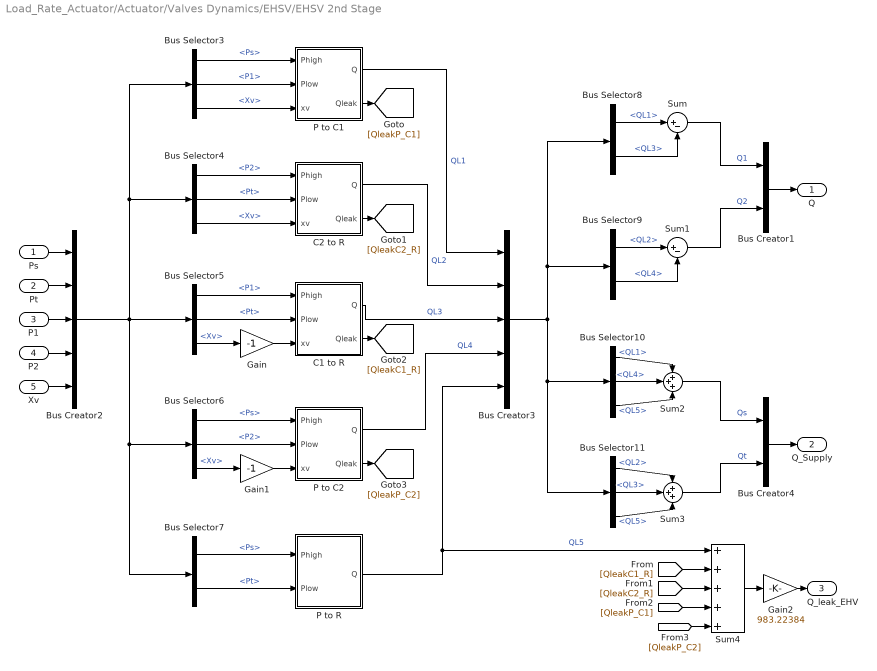
== system Load_Rate_Actuator/Actuator/Valves Dynamics/EHSV/EHSV 2nd Stage ==
  Ps : Inport
  Pt : Inport  Port=2
  P1 : Inport  Port=3
  P2 : Inport  Port=4
  Xv : Inport  Port=5
  Bus Creator1 : BusCreator  Inputs=2
  Bus Creator2 : BusCreator  Inputs=5
  Bus Creator3 : BusCreator  Inputs=5
  Bus Creator4 : BusCreator  Inputs=2
  Bus Selector10 : BusSelector  OutputSignals=QL1,QL4,QL5
  Bus Selector11 : BusSelector  OutputSignals=QL2,QL3,QL5
  Bus Selector3 : BusSelector  OutputSignals=Ps,P1,Xv
  Bus Selector4 : BusSelector  OutputSignals=P2,Pt,Xv
  Bus Selector5 : BusSelector  OutputSignals=P1,Pt,Xv
  Bus Selector6 : BusSelector  OutputSignals=Ps,P2,Xv
  Bus Selector7 : BusSelector  OutputSignals=Ps,Pt
  Bus Selector8 : BusSelector  OutputSignals=QL1,QL3
  Bus Selector9 : BusSelector  OutputSignals=QL2,QL4
  C1 to R : Subsystem
  C2 to R : Subsystem
  Gain : Gain  Gain=-1
  Gain1 : Gain  Gain=-1
  Gain2 : Gain  Gain=983.22384
  P to C1 : Subsystem
  P to C2 : Subsystem
  P to R : Subsystem
  Sum : Sum  Inputs=|+-
  Sum1 : Sum  Inputs=|+-
  Sum2 : Sum  Inputs=+++
  Sum3 : Sum  Inputs=+++
  Sum4 : Sum  Inputs=+++++
  Q : Outport
  Q_Supply : Outport  Port=2
  Q_leak_EHV : Outport  Port=3
  wires:
  Bus Creator1/1 -> Q/1
  Bus Selector3/1 -> P to C1/1(Phigh)  "<Ps>"
  Bus Selector3/2 -> P to C1/2(Plow)  "<P1>"
  Bus Selector3/3 -> P to C1/3(xv)  "<Xv>"
  Bus Selector4/1 -> C2 to R/1(Phigh)  "<P2>"
  Bus Selector4/2 -> C2 to R/2(Plow)  "<Pt>"
  Bus Selector4/3 -> C2 to R/3(xv)  "<Xv>"
  Bus Selector5/3 -> Gain/1  "<Xv>"
  Bus Selector6/1 -> P to C2/1(Phigh)  "<Ps>"
  Bus Selector6/2 -> P to C2/2(Plow)  "<P2>"
  Bus Selector6/3 -> Gain1/1  "<Xv>"
  Bus Selector7/1 -> P to R/1(Phigh)  "<Ps>"
  Bus Selector7/2 -> P to R/2(Plow)  "<Pt>"
  Bus Selector5/1 -> C1 to R/1(Phigh)  "<P1>"
  Bus Selector5/2 -> C1 to R/2(Plow)  "<Pt>"
  P to C1/1(Q) -> Bus Creator3/1  "QL1"
  C2 to R/1(Q) -> Bus Creator3/2  "QL2"
  C1 to R/1(Q) -> Bus Creator3/3  "QL3"
  P to C2/1(Q) -> Bus Creator3/4  "QL4"
  P to R/1(Q) -> Sum4/1, Bus Creator3/5  "QL5"
  Bus Creator2/1 -> Bus Selector5/1, Bus Selector3/1, Bus Selector4/1, Bus Selector7/1, Bus Selector6/1
  Bus Selector8/1 -> Sum/1  "<QL1>"
  Bus Selector8/2 -> Sum/2  "<QL3>"
  Bus Selector9/1 -> Sum1/1  "<QL2>"
  Bus Selector9/2 -> Sum1/2  "<QL4>"
  Bus Selector10/1 -> Sum2/1  "<QL1>"
  Bus Selector10/2 -> Sum2/2  "<QL4>"
  Bus Selector10/3 -> Sum2/3  "<QL5>"
  Bus Selector11/1 -> Sum3/1  "<QL2>"
  Bus Selector11/2 -> Sum3/2  "<QL3>"
  Bus Selector11/3 -> Sum3/3  "<QL5>"
  Bus Creator4/1 -> Q_Supply/1
  Bus Creator3/1 -> Bus Selector8/1, Bus Selector9/1, Bus Selector11/1, Bus Selector10/1
  Sum/1 -> Bus Creator1/1  "Q1"
  Sum1/1 -> Bus Creator1/2  "Q2"
  Sum2/1 -> Bus Creator4/1  "Qs"
  Sum3/1 -> Bus Creator4/2  "Qt"
  Ps/1 -> Bus Creator2/1
  Pt/1 -> Bus Creator2/2
  P1/1 -> Bus Creator2/3
  P2/1 -> Bus Creator2/4
  Xv/1 -> Bus Creator2/5
  Gain/1 -> C1 to R/3(xv)
  Gain1/1 -> P to C2/3(xv)
  Sum4/1 -> Gain2/1
  P to C1/2(Qleak) -> [QleakP_C1]
  C2 to R/2(Qleak) -> [QleakC2_R]
  C1 to R/2(Qleak) -> [QleakC1_R]
  P to C2/2(Qleak) -> [QleakP_C2]
  [QleakC1_R] -> Sum4/2
  [QleakC2_R] -> Sum4/3
  [QleakP_C2] -> Sum4/5
  [QleakP_C1] -> Sum4/4
  Gain2/1 -> Q_leak_EHV/1

== system Load_Rate_Actuator/Actuator/Valves Dynamics/EHSV/EHSV Test ==
  In1 : Inport
  Constant1 : Constant  Value=EHSVTest.Enable
  Constant3 : Constant  Value=1500
  EHVS freq test Selector1 : MultiPortSwitch
  Out1 : Outport
  wires:
  Constant1/1 -> EHVS freq test Selector1/1
  EHVS freq test Selector1/1 -> Out1/1
  In1/1 -> EHVS freq test Selector1/4, EHVS freq test Selector1/2
  Constant3/1 -> EHVS freq test Selector1/3

== system Load_Rate_Actuator/Actuator/Valves Dynamics/EHSV/EHSV Test1 ==
  In1 : Inport
  Constant1 : Constant  Value=EHSVTest.Enable
  Constant3 : Constant  Value=1500
  EHVS freq test Selector1 : MultiPortSwitch
  Out1 : Outport
  wires:
  Constant1/1 -> EHVS freq test Selector1/1
  EHVS freq test Selector1/1 -> Out1/1
  In1/1 -> EHVS freq test Selector1/4, EHVS freq test Selector1/2
  Constant3/1 -> EHVS freq test Selector1/3

== system Load_Rate_Actuator/Actuator/Valves Dynamics/EHSV/EHSV Test2 ==
  In1 : Inport
  Constant1 : Constant  Value=EHSVTest.Enable
  Constant3 : Constant  Value=3000
  EHVS freq test Selector1 : MultiPortSwitch
  Out1 : Outport
  wires:
  Constant1/1 -> EHVS freq test Selector1/1
  EHVS freq test Selector1/1 -> Out1/1
  In1/1 -> EHVS freq test Selector1/4, EHVS freq test Selector1/2
  Constant3/1 -> EHVS freq test Selector1/3

== system Load_Rate_Actuator/Actuator/Valves Dynamics/EHSV/EHSV Test3 ==
  In1 : Inport
  Constant1 : Constant  Value=EHSVTest.Enable
  Constant3 : Constant  Value=0
  EHVS freq test Selector1 : MultiPortSwitch
  Out1 : Outport
  wires:
  Constant1/1 -> EHVS freq test Selector1/1
  EHVS freq test Selector1/1 -> Out1/1
  In1/1 -> EHVS freq test Selector1/4, EHVS freq test Selector1/2
  Constant3/1 -> EHVS freq test Selector1/3

== system Load_Rate_Actuator/Actuator/Valves Dynamics/EHSV/EHSV input ==
  CurrentCmd : Inport
  Constant : Constant  Value=EHSVTest.Enable
  EHSV Freq Test : Sin  Amplitude=EHSVFreqTest.Sine.Amplitude  Bias=EHSVFreqTest.Sine.Bias  Frequency=EHSVFreqTest.Sine.Frequency  SampleTime=0
  EHVS freq test Selector : MultiPortSwitch
  Step : Step  Time=EHSV.Step.Time  After=EHSV.Step.Value  SampleTime=0
  EHSV_current : Outport
  wires:
  Constant/1 -> EHVS freq test Selector/1
  EHSV Freq Test/1 -> EHVS freq test Selector/3
  Step/1 -> EHVS freq test Selector/4
  EHVS freq test Selector/1 -> EHSV_current/1  "EHSV_current_cmd"
  CurrentCmd/1 -> EHVS freq test Selector/2

== system Load_Rate_Actuator/Actuator/Valves Dynamics/Inlet Check Valve/Inlet Check Valve Flow ==
  P1 : Inport
  P2 : Inport  Port=2
  Abs : Abs
  Constant : Constant  Value=Acv*sqrt(2/Rho)
  Constant1 : Constant  Value=Pcvi
  Gain : Gain  Gain=Cd/Pcvi
  Math Function : Math  Operator=sqrt  SaturateOnIntegerOverflow=on
  Product : Product  RndMeth=Zero
  Product1 : Product  RndMeth=Zero
  Product2 : Product  RndMeth=Zero
  Saturation : Saturate  UpperLimit=Cd  LowerLimit=0
  Sign : Signum
  Sum : Sum  Inputs=|+-
  Sum1 : Sum  Inputs=|+-
  Q : Outport
  wires:
  P1/1 -> Sum/1
  P2/1 -> Sum/2
  Sum/1 -> Sum1/1, Abs/1, Sign/1
  Constant1/1 -> Sum1/2
  Sum1/1 -> Gain/1
  Gain/1 -> Saturation/1
  Saturation/1 -> Product/1
  Constant/1 -> Product/2
  Abs/1 -> Math Function/1
  Sign/1 -> Product1/1
  Math Function/1 -> Product1/2
  Product1/1 -> Product2/1
  Product/1 -> Product2/2
  Product2/1 -> Q/1

== system Load_Rate_Actuator/Actuator/Valves Dynamics/Return Check Valve/Return Check Valve Flow ==
  P1 : Inport
  P2 : Inport  Port=2
  Abs : Abs
  Constant : Constant  Value=Acv*sqrt(2/Rho)
  Constant1 : Constant  Value=Pcvr
  Gain : Gain  Gain=Cd/Pcvr
  Math Function : Math  Operator=sqrt  SaturateOnIntegerOverflow=on
  Product : Product  RndMeth=Zero
  Product1 : Product  RndMeth=Zero
  Product2 : Product  RndMeth=Zero
  Saturation : Saturate  UpperLimit=Cd  LowerLimit=0
  Sign : Signum
  Sum : Sum  Inputs=|-+
  Sum1 : Sum  Inputs=|+-
  Q : Outport
  wires:
  P1/1 -> Sum/1
  P2/1 -> Sum/2
  Sum/1 -> Sum1/1, Abs/1, Sign/1
  Constant1/1 -> Sum1/2
  Sum1/1 -> Gain/1
  Gain/1 -> Saturation/1
  Saturation/1 -> Product/1
  Constant/1 -> Product/2
  Abs/1 -> Math Function/1
  Sign/1 -> Product1/1
  Math Function/1 -> Product1/2
  Product1/1 -> Product2/1
  Product/1 -> Product2/2
  Product2/1 -> Q/1

== system Load_Rate_Actuator/Actuator/Cylinder Dynamics/Piston Dynamics/Seal Friction Force/Force friction 2 Rod backup + scrapper seal ==
  Pressure : Inport
  Ar : Gain  Gain=Ar_seal
  Fc+Fh2 : Sum
  Friction - O-ring compression1 : Lookup_n-D  BreakpointsForDimension1=[0,5,10,15,20,25]  BreakpointsForDimension2=[70,80,90]  IndexSearchMethod=Linear search  Table=reshape([0,0.3,0.65,0.97313,1.37,1.7,0,0.6,1.22,1.82,2.45,3.05,0,0.8,1.6,2.37,3.2,3.98],6,3)  RndMeth=Simplest  InputSameDT=on
  Friction - O-ring hydraulic pressure1 : Lookup_n-D  NumberOfTableDimensions=1  BreakpointsForDimension1=|  BreakpointsForDimension2=[70,80,90]  IndexSearchMethod=Linear search  Table=|  RndMeth=Simplest  InputSameDT=on
      BreakpointsForDimension1=|
      | [0
      | 500
      | 1000
      | 1500
      | 2000
      | 2500
      | 3000]
      Table=|
      | [0
      | 24.5
      | 37.5
      | 48
      | 58
      | 67
      | 72.1]
  Lr : Gain  Gain=Lr_seal
  Seal compression : Constant  Value=seal_compression
  Seal hardness : Constant  Value=seal_hardness
  Ffriction : Outport
  wires:
  Friction - O-ring compression1/1 -> Lr/1
  Lr/1 -> Fc+Fh2/2  "Fc"
  Pressure/1 -> Friction - O-ring hydraulic pressure1/1
  Friction - O-ring hydraulic pressure1/1 -> Ar/1
  Ar/1 -> Fc+Fh2/1  "Fh"
  Fc+Fh2/1 -> Ffriction/1
  Seal compression/1 -> [Seal_compression]
  [Seal_compression] -> Friction - O-ring compression1/1
  Seal hardness/1 -> [Seal_hardness]
  [Seal_hardness] -> Friction - O-ring compression1/2

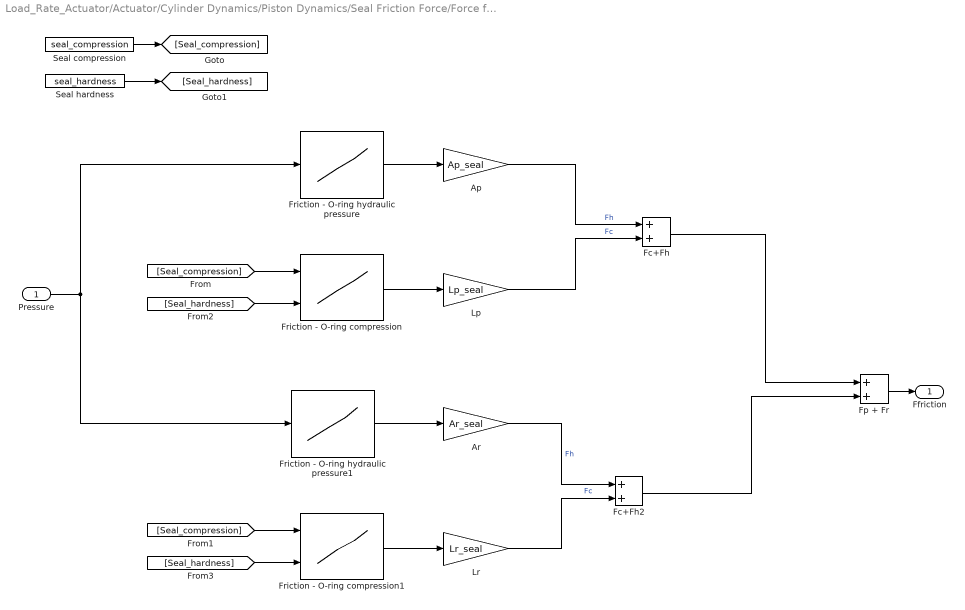
== system Load_Rate_Actuator/Actuator/Cylinder Dynamics/Piston Dynamics/Seal Friction Force/Force friction Piston+rod extension ==
  Pressure : Inport
  Ap : Gain  Gain=Ap_seal
  Ar : Gain  Gain=Ar_seal
  Fc+Fh : Sum
  Fc+Fh2 : Sum
  Fp + Fr : Sum
  Friction - O-ring compression : Lookup_n-D  BreakpointsForDimension1=[0,5,10,15,20,25]  BreakpointsForDimension2=[70,80,90]  IndexSearchMethod=Linear search  Table=reshape([0,0.3,0.65,0.97313,1.37,1.7,0,0.6,1.22,1.82,2.45,3.05,0,0.8,1.6,2.37,3.2,3.98],6,3)  RndMeth=Simplest  InputSameDT=on
  Friction - O-ring compression1 : Lookup_n-D  BreakpointsForDimension1=[0,5,10,15,20,25]  BreakpointsForDimension2=[70,80,90]  IndexSearchMethod=Linear search  Table=reshape([0,0.3,0.65,0.97313,1.37,1.7,0,0.6,1.22,1.82,2.45,3.05,0,0.8,1.6,2.37,3.2,3.98],6,3)  RndMeth=Simplest  InputSameDT=on
  Friction - O-ring hydraulic pressure : Lookup_n-D  NumberOfTableDimensions=1  BreakpointsForDimension1=|  BreakpointsForDimension2=[70,80,90]  IndexSearchMethod=Linear search  Table=|  RndMeth=Simplest  InputSameDT=on
      BreakpointsForDimension1=|
      | [0
      | 500
      | 1000
      | 1500
      | 2000
      | 2500
      | 3000]
      Table=|
      | [0
      | 24.5
      | 37.5
      | 48
      | 58
      | 67
      | 72.1]
  Friction - O-ring hydraulic pressure1 : Lookup_n-D  NumberOfTableDimensions=1  BreakpointsForDimension1=|  BreakpointsForDimension2=[70,80,90]  IndexSearchMethod=Linear search  Table=|  RndMeth=Simplest  InputSameDT=on
      BreakpointsForDimension1=|
      | [0
      | 500
      | 1000
      | 1500
      | 2000
      | 2500
      | 3000]
      Table=|
      | [0
      | 24.5
      | 37.5
      | 48
      | 58
      | 67
      | 72.1]
  Lp : Gain  Gain=Lp_seal
  Lr : Gain  Gain=Lr_seal
  Seal compression : Constant  Value=seal_compression
  Seal hardness : Constant  Value=seal_hardness
  Ffriction : Outport
  wires:
  Friction - O-ring compression/1 -> Lp/1
  Lp/1 -> Fc+Fh/2  "Fc"
  Friction - O-ring hydraulic pressure/1 -> Ap/1
  Ap/1 -> Fc+Fh/1  "Fh"
  Fp + Fr/1 -> Ffriction/1
  Friction - O-ring compression1/1 -> Lr/1
  Lr/1 -> Fc+Fh2/2  "Fc"
  Pressure/1 -> Friction - O-ring hydraulic pressure/1, Friction - O-ring hydraulic pressure1/1
  Friction - O-ring hydraulic pressure1/1 -> Ar/1
  Ar/1 -> Fc+Fh2/1  "Fh"
  Fc+Fh2/1 -> Fp + Fr/2
  Fc+Fh/1 -> Fp + Fr/1
  Seal compression/1 -> [Seal_compression]
  [Seal_compression] -> Friction - O-ring compression/1
  [Seal_compression] -> Friction - O-ring compression1/1
  Seal hardness/1 -> [Seal_hardness]
  [Seal_hardness] -> Friction - O-ring compression/2
  [Seal_hardness] -> Friction - O-ring compression1/2

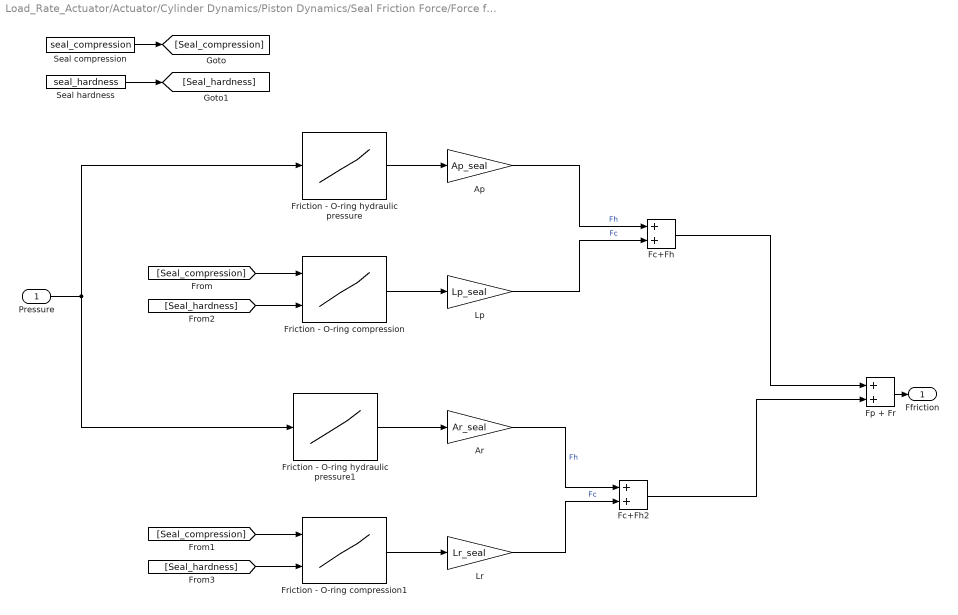
== system Load_Rate_Actuator/Actuator/Cylinder Dynamics/Piston Dynamics/Seal Friction Force/Force friction Piston+rod retraction ==
  Pressure : Inport
  Ap : Gain  Gain=Ap_seal
  Ar : Gain  Gain=Ar_seal
  Fc+Fh : Sum
  Fc+Fh2 : Sum
  Fp + Fr : Sum
  Friction - O-ring compression : Lookup_n-D  BreakpointsForDimension1=[0,5,10,15,20,25]  BreakpointsForDimension2=[70,80,90]  IndexSearchMethod=Linear search  Table=reshape([0,0.3,0.65,0.97313,1.37,1.7,0,0.6,1.22,1.82,2.45,3.05,0,0.8,1.6,2.37,3.2,3.98],6,3)  RndMeth=Simplest  InputSameDT=on
  Friction - O-ring compression1 : Lookup_n-D  BreakpointsForDimension1=[0,5,10,15,20,25]  BreakpointsForDimension2=[70,80,90]  IndexSearchMethod=Linear search  Table=reshape([0,0.3,0.65,0.97313,1.37,1.7,0,0.6,1.22,1.82,2.45,3.05,0,0.8,1.6,2.37,3.2,3.98],6,3)  RndMeth=Simplest  InputSameDT=on
  Friction - O-ring hydraulic pressure : Lookup_n-D  NumberOfTableDimensions=1  BreakpointsForDimension1=|  BreakpointsForDimension2=[70,80,90]  IndexSearchMethod=Linear search  Table=|  RndMeth=Simplest  InputSameDT=on
      BreakpointsForDimension1=|
      | [0
      | 500
      | 1000
      | 1500
      | 2000
      | 2500
      | 3000]
      Table=|
      | [0
      | 24.5
      | 37.5
      | 48
      | 58
      | 67
      | 72.1]
  Friction - O-ring hydraulic pressure1 : Lookup_n-D  NumberOfTableDimensions=1  BreakpointsForDimension1=|  BreakpointsForDimension2=[70,80,90]  IndexSearchMethod=Linear search  Table=|  RndMeth=Simplest  InputSameDT=on
      BreakpointsForDimension1=|
      | [0
      | 500
      | 1000
      | 1500
      | 2000
      | 2500
      | 3000]
      Table=|
      | [0
      | 24.5
      | 37.5
      | 48
      | 58
      | 67
      | 72.1]
  Lp : Gain  Gain=Lp_seal
  Lr : Gain  Gain=Lr_seal
  Seal compression : Constant  Value=seal_compression
  Seal hardness : Constant  Value=seal_hardness
  Ffriction : Outport
  wires:
  Friction - O-ring compression/1 -> Lp/1
  Lp/1 -> Fc+Fh/2  "Fc"
  Friction - O-ring hydraulic pressure/1 -> Ap/1
  Ap/1 -> Fc+Fh/1  "Fh"
  Fp + Fr/1 -> Ffriction/1
  Friction - O-ring compression1/1 -> Lr/1
  Lr/1 -> Fc+Fh2/2  "Fc"
  Pressure/1 -> Friction - O-ring hydraulic pressure/1, Friction - O-ring hydraulic pressure1/1
  Friction - O-ring hydraulic pressure1/1 -> Ar/1
  Ar/1 -> Fc+Fh2/1  "Fh"
  Fc+Fh2/1 -> Fp + Fr/2
  Fc+Fh/1 -> Fp + Fr/1
  Seal compression/1 -> [Seal_compression]
  [Seal_compression] -> Friction - O-ring compression/1
  [Seal_compression] -> Friction - O-ring compression1/1
  Seal hardness/1 -> [Seal_hardness]
  [Seal_hardness] -> Friction - O-ring compression/2
  [Seal_hardness] -> Friction - O-ring compression1/2

== system Load_Rate_Actuator/Actuator/Cylinder Dynamics/Piston Dynamics/Seal Friction Force/Stribeck effect ==
  Xp : Inport
  Abs : Abs
  Backlash : Backlash  BacklashWidth=.1
  Divide : Product  Inputs=*/
  Fcn : Fcn  Expr=exp(-u/frictionstribeck_velocity)
  Manual Switch : ManualSwitch  CurrentSetting=0
  Manual Switch1 : ManualSwitch  CurrentSetting=0
  Product : Product  RndMeth=Zero
  Stribeck factor : Outport
  wires:
  Xp/1 -> Manual Switch1/1, Backlash/1
  Abs/1 -> Divide/1, Fcn/1
  Fcn/1 -> Manual Switch/2, Product/2
  Divide/1 -> Product/1
  Product/1 -> Manual Switch/1
  Manual Switch/1 -> Stribeck factor/1
  Manual Switch1/1 -> Divide/2, Abs/1
  Backlash/1 -> Manual Switch1/2

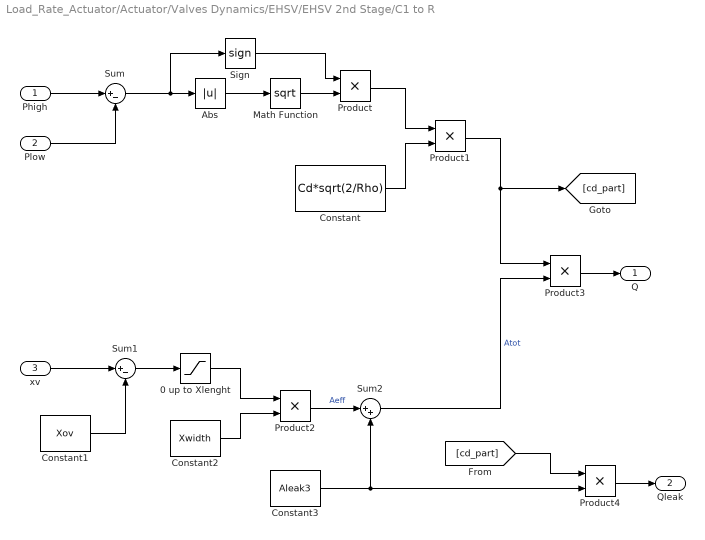
== system Load_Rate_Actuator/Actuator/Valves Dynamics/EHSV/EHSV 2nd Stage/C1 to R ==
  Phigh : Inport
  Plow : Inport  Port=2
  xv : Inport  Port=3
  0 up to Xlenght : Saturate  UpperLimit=Xlength  LowerLimit=0
  Abs : Abs
  Constant : Constant  Value=Cd*sqrt(2/Rho)
  Constant1 : Constant  Value=Xov
  Constant2 : Constant  Value=Xwidth
  Constant3 : Constant  Value=Aleak3
  Math Function : Math  Operator=sqrt  SaturateOnIntegerOverflow=on
  Product{,1..4} (5 alike) : Product  RndMeth=Zero
  Sign : Signum
  Sum : Sum  Inputs=|+-
  Sum1 : Sum  Inputs=|+-
  Sum2 : Sum  Inputs=|++
  Q : Outport
  Qleak : Outport  Port=2
  wires:
  Phigh/1 -> Sum/1
  Plow/1 -> Sum/2
  Sum/1 -> Abs/1, Sign/1
  Abs/1 -> Math Function/1
  Sign/1 -> Product/1
  Math Function/1 -> Product/2
  Constant/1 -> Product1/2
  Product/1 -> Product1/1
  xv/1 -> Sum1/1
  Constant1/1 -> Sum1/2
  Sum1/1 -> 0 up to Xlenght/1
  0 up to Xlenght/1 -> Product2/1
  Constant2/1 -> Product2/2
  Product2/1 -> Sum2/1  "Aeff"
  Constant3/1 -> Product4/2, Sum2/2
  Product1/1 -> [cd_part], Product3/1
  Sum2/1 -> Product3/2  "Atot"
  Product3/1 -> Q/1
  Product4/1 -> Qleak/1
  [cd_part] -> Product4/1

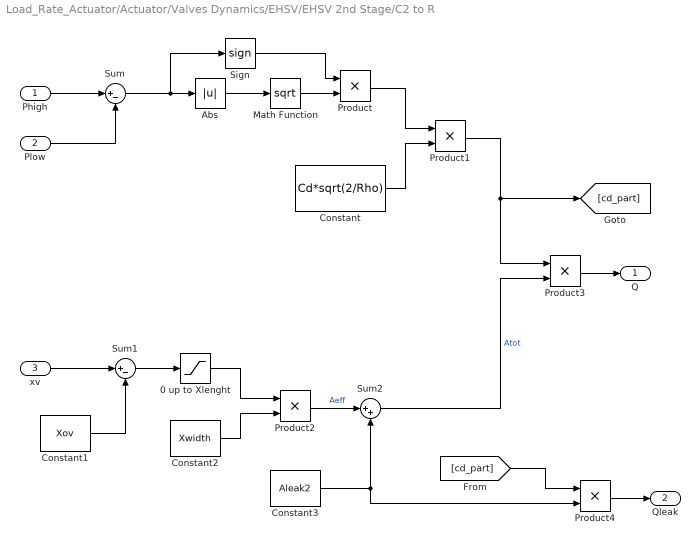
== system Load_Rate_Actuator/Actuator/Valves Dynamics/EHSV/EHSV 2nd Stage/C2 to R ==
  Phigh : Inport
  Plow : Inport  Port=2
  xv : Inport  Port=3
  0 up to Xlenght : Saturate  UpperLimit=Xlength  LowerLimit=0
  Abs : Abs
  Constant : Constant  Value=Cd*sqrt(2/Rho)
  Constant1 : Constant  Value=Xov
  Constant2 : Constant  Value=Xwidth
  Constant3 : Constant  Value=Aleak2
  Math Function : Math  Operator=sqrt  SaturateOnIntegerOverflow=on
  Product{,1..4} (5 alike) : Product  RndMeth=Zero
  Sign : Signum
  Sum : Sum  Inputs=|+-
  Sum1 : Sum  Inputs=|+-
  Sum2 : Sum  Inputs=|++
  Q : Outport
  Qleak : Outport  Port=2
  wires:
  Product3/1 -> Q/1
  Sum2/1 -> Product3/2  "Atot"
  Product1/1 -> [cd_part], Product3/1
  Product2/1 -> Sum2/1  "Aeff"
  Constant2/1 -> Product2/2
  0 up to Xlenght/1 -> Product2/1
  Sum1/1 -> 0 up to Xlenght/1
  Constant1/1 -> Sum1/2
  xv/1 -> Sum1/1
  Product/1 -> Product1/1
  Constant/1 -> Product1/2
  Math Function/1 -> Product/2
  Sign/1 -> Product/1
  Abs/1 -> Math Function/1
  Sum/1 -> Sign/1, Abs/1
  Plow/1 -> Sum/2
  Phigh/1 -> Sum/1
  Constant3/1 -> Product4/2, Sum2/2
  Product4/1 -> Qleak/1
  [cd_part] -> Product4/1
